simulink model "FM_10_Controle_LQR"  (Simulink 7.1)
settings: Solver=ode45  StartTime=0.0  StopTime=300  RelTol=1e-3
undefined symbols (not defined in the file or in its folder): analoginput, analogoutput, QT
libraries: daqlib x2, simulink x1
settings Model: Creator=didaticontrol  LastModifiedBy=didaticontrol

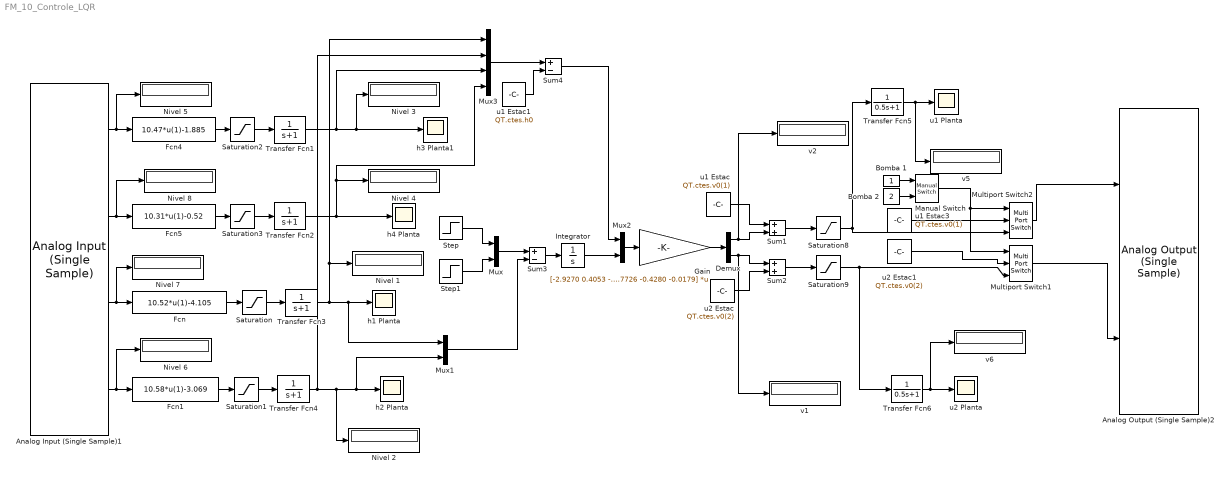
== system FM_10_Controle_LQR ==
  Analog Input (Single Sample)1 : daqlib/Analog Input (Single Sample)  DialogController=daqcreatedialog  DialogControllerArgs=DataTag0  DeviceMenu=nidaq Dev1 (USB-6008)  Device=nidaq Dev1 (USB-6008)  ObjConstructor=analoginput('nidaq','Dev1')  InputType=Differential  NChannelsSelected=4  Channels=1$0$$5$#1$1$$5$#1$2$$5$#1$3$$5$#  NPorts=1 per hardware channel  BlockSampleTime=10e-3
  Analog Output (Single Sample)2 : daqlib/Analog Output (Single Sample)  DialogController=daqcreatedialog  DialogControllerArgs=DataTag1  DeviceMenu=nidaq Dev1 (USB-6008)  Device=nidaq Dev1 (USB-6008)  ObjConstructor=analogoutput('nidaq','Dev1')  NChannelsSelected=2  Channels=1$0$$1$0$#1$1$$1$0$#  NPorts=1 per hardware channel
  Bomba 1 : Constant
  Bomba 2 : Constant  Value=2
  Demux : Demux  Outputs=2
  Fcn : Fcn  Expr=10.52*u(1)-4.105  SampleTime=10e-3
  Fcn1 : Fcn  Expr=10.58*u(1)-3.069
  Fcn4 : Fcn  Expr=10.47*u(1)-1.885
  Fcn5 : Fcn  Expr=10.31*u(1)-0.52
  Gain : Gain  Gain=[-2.9270 0.4053 -0.1281 4.2779 0.1321 -0.0683;9.4117 0.0732 0.4042 -3.7726 -0.4280 -0.0179]  Multiplication=Matrix(K*u)  ParameterDataType=sfix(16)  ParameterScaling=2^0  OutDataType=sfix(16)  OutScaling=2^0
  Integrator : Integrator  LimitOutput=on
  Manual Switch : simulink/Signal Routing/Manual Switch  SystemSampleTime=-1  sw=1  action=0  varsize=off
  Multiport Switch1 : MultiPortSwitch  Inputs=2  OutDataType=sfix(16)  OutScaling=2^0
  Multiport Switch2 : MultiPortSwitch  Inputs=2  OutDataType=sfix(16)  OutScaling=2^0
  Mux : Mux  Inputs=2
  Mux1 : Mux  Inputs=2
  Mux2 : Mux  Inputs=2
  Mux3 : Mux
  Nivel {1..8} (8 alike) : Display
  Saturation : Saturate  UpperLimit=23  LowerLimit=0  SampleTime=10e-3
  Saturation1 : Saturate  UpperLimit=23  LowerLimit=0
  Saturation2 : Saturate  UpperLimit=23  LowerLimit=0
  Saturation3 : Saturate  UpperLimit=23  LowerLimit=0
  Saturation8 : Saturate  UpperLimit=0.7*5  LowerLimit=0  SampleTime=10e-3
  Saturation9 : Saturate  UpperLimit=0.7*5  LowerLimit=0  SampleTime=10e-3
  Step : Step  Time=100  Before=QT.ctes.h0(1)  After=QT.ctes.h0(1)+1  SampleTime=0
  Step1 : Step  Time=200  Before=QT.ctes.h0(2)  After=QT.ctes.h0(2)+1  SampleTime=0
  Sum1 : Sum  OutDataType=sfix(16)  OutScaling=2^0
  Sum2 : Sum  OutDataType=sfix(16)  OutScaling=2^0
  Sum3 : Sum  Inputs=+-  OutDataType=sfix(16)  OutScaling=2^0
  Sum4 : Sum  Inputs=+-  OutDataType=sfix(16)  OutScaling=2^0
  Transfer Fcn{1..4} (4 alike) : TransferFcn  Denominator=[1 1]
  Transfer Fcn5 : TransferFcn  Denominator=[0.5 1]
  Transfer Fcn6 : TransferFcn  Denominator=[0.5 1]
  h1 Planta : Scope
      settings: YMin=0  YMax=8  SaveName=h1_real
  h2 Planta : Scope
      settings: YMin=0  YMax=12  SaveName=h2_real
  h3 Planta1 : Scope
      settings: YMin=0  YMax=8  SaveName=h3_real
  h4 Planta : Scope
      settings: YMin=0  YMax=17  SaveName=h4_real
  u1 Planta : Scope
      settings: YMin=1.4  YMax=3.5  SaveName=u1_real
  u1 Estac : Constant  Value=QT.ctes.v0(1)
  u1 Estac1 : Constant  Value=QT.ctes.h0
  u1 Estac3 : Constant  Value=QT.ctes.v0(1)
  u2 Planta : Scope
      settings: YMin=0  YMax=3.5  SaveName=u2_real
  u2 Estac : Constant  Value=QT.ctes.v0(2)
  u2 Estac1 : Constant  Value=QT.ctes.v0(2)
  v{1..2,5..6} (4 alike) : Display
  wires:
  Analog Input (Single Sample)1/3 -> Fcn/1, Nivel 7/1
  Fcn/1 -> Saturation/1
  Fcn1/1 -> Saturation1/1
  Analog Input (Single Sample)1/4 -> Fcn1/1, Nivel 6/1
  Analog Input (Single Sample)1/2 -> Fcn5/1, Nivel 8/1
  Analog Input (Single Sample)1/1 -> Nivel 5/1, Fcn4/1
  Fcn4/1 -> Saturation2/1
  Fcn5/1 -> Saturation3/1
  Saturation8/1 -> Transfer Fcn5/1, Multiport Switch2/3
  Saturation9/1 -> Transfer Fcn6/1, Multiport Switch1/3
  Sum1/1 -> Saturation8/1
  u1 Estac/1 -> Sum1/1
  Sum2/1 -> Saturation9/1
  u2 Estac/1 -> Sum2/2
  Step/1 -> Mux/1
  Step1/1 -> Mux/2
  Mux/1 -> Sum3/1
  Sum3/1 -> Integrator/1
  Mux2/1 -> Gain/1
  Gain/1 -> Demux/1
  Demux/1 -> Sum1/2, v2/1
  Demux/2 -> Sum2/1, v1/1
  Saturation2/1 -> Transfer Fcn1/1
  Transfer Fcn1/1 -> Mux3/3, h3 Planta1/1, Nivel 3/1
  Saturation3/1 -> Transfer Fcn2/1
  Transfer Fcn2/1 -> h4 Planta/1, Nivel 4/1, Mux3/4
  Saturation/1 -> Transfer Fcn3/1
  Transfer Fcn3/1 -> Nivel 1/1, Mux3/1, h1 Planta/1, Mux1/1
  Saturation1/1 -> Transfer Fcn4/1
  Transfer Fcn4/1 -> Nivel 2/1, h2 Planta/1, Mux1/2, Mux3/2
  Transfer Fcn6/1 -> u2 Planta/1, v6/1
  Transfer Fcn5/1 -> u1 Planta/1, v5/1
  Multiport Switch1/1 -> Analog Output (Single Sample)2/2
  Multiport Switch2/1 -> Analog Output (Single Sample)2/1
  Bomba 1/1 -> Manual Switch/1
  Bomba 2/1 -> Manual Switch/2
  Manual Switch/1 -> Multiport Switch2/1, Multiport Switch1/1
  Mux3/1 -> Sum4/1
  Sum4/1 -> Mux2/1
  u1 Estac1/1 -> Sum4/2
  u1 Estac3/1 -> Multiport Switch2/2
  u2 Estac1/1 -> Multiport Switch1/2
  Mux1/1 -> Sum3/2
  Integrator/1 -> Mux2/2
